simulink model "mamdani_25_rules_trimf_centroid_squarewave"  (R2016b)
settings: Solver=ode45  StartTime=0.0  StopTime=1000  RelTol=1e-3  EnableMultiTasking=on
libraries: fuzblock x1
settings Model: ModifiedByFormat=adolfo  Creator=adolfo  LastModifiedBy=adolfo
settings SolverCC: ZeroCrossControl=DisableAll  ZeroCrossAlgorithm=Adaptive
settings DataIOCC: LimitDataPoints=on  SaveFormat=Array
settings OptimizationCC: LifeSpan=inf
settings DebuggingCC: SolverPrmCheckMsg=warning  SFUnexpectedBacktrackingDiag=warning  SFNoUnconditionalDefaultTransitionDiag=warning  SFExecutionAtInitializationDiag=none
settings HardwareCC: ProdBitPerPointer=32  ProdBitPerSizeT=32  ProdBitPerPtrDiffT=32  ProdLargestAtomicFloat=None  ProdIntDivRoundTo=Undefined  ProdEndianess=Unspecified  ProdWordSize=32  ProdHWDeviceType=32-bit Generic
settings ModelReferenceCC: PropagateSignalLabelsOutOfModel=off
settings GRTTargetCC: TargetLangStandard=C89/C90 (ANSI)  GeneratePreprocessorConditionals=Disable all
settings ConfigComp: CovMetricSettings=dw  CovHtmlReporting=on  CovSaveCumulativeToWorkspaceVar=on  CovSaveSingleToWorkspaceVar=on  CovExternalEMLEnable=off  CovSFcnEnable=off

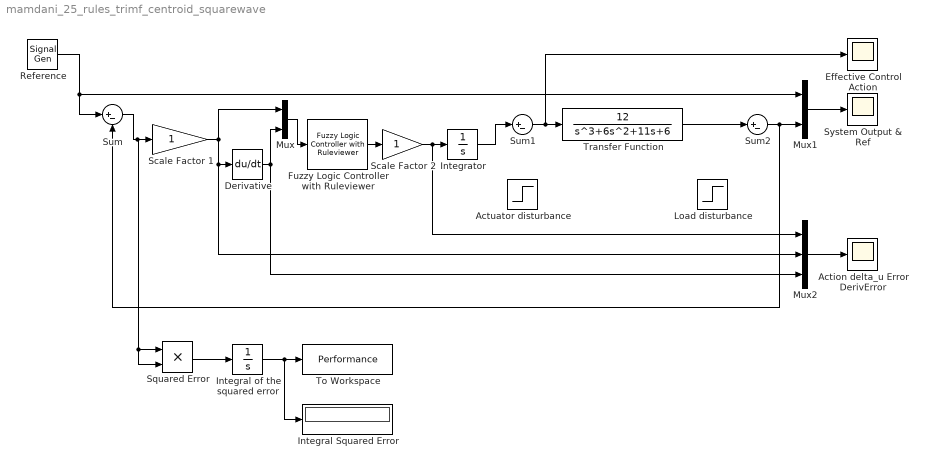
== system mamdani_25_rules_trimf_centroid_squarewave ==
  Action delta_u Error DerivError : Scope
  "Actuator disturbance " : Step  SampleTime=0
  Derivative : Derivative
  "Effective Control Action " : Scope
  Fuzzy Logic Controller with Ruleviewer : fuzblock/Fuzzy Logic  Controller  with Ruleviewer  fismatrix=mamdani_25_rules_trimf_centroid  Ts=1
  "Integral Squared Error " : Display
  "Integral of the squared error " : Integrator
  Integrator : Integrator
  Load disturbance : Step  SampleTime=0
  Mux : Mux  Inputs=2
  Mux1 : Mux  Inputs=2
  Mux2 : Mux  Inputs=3
  Reference : SignalGenerator  WaveForm=square  Amplitude=-1  Frequency=0.01  Units=rad/sec
  Scale Factor 1 : Gain
  Scale Factor 2 : Gain
  Squared Error : Product
  Sum : Sum  Inputs=|+-
  Sum1 : Sum  Inputs=|+-
  Sum2 : Sum  Inputs=|+-
  System Output & Ref : Scope
  To Workspace : ToWorkspace  VariableName=Performance  SaveFormat=Timeseries  SampleTime=-1
  Transfer Function : TransferFcn  Numerator=[12]  Denominator=[1 6 11 6]
  wires:
  Reference/1 -> Sum/1, Mux1/1
  Sum/1 -> Squared Error/2, Squared Error/1, Scale Factor 1/1
  Derivative/1 -> Mux2/3, Mux/2
  Scale Factor 1/1 -> Mux/1, Mux2/2, Derivative/1
  Scale Factor 2/1 -> Mux2/1, Integrator/1
  Integrator/1 -> Sum1/1
  Sum1/1 -> "Effective Control Action "/1, Transfer Function/1
  Transfer Function/1 -> Sum2/1
  Sum2/1 -> Sum/2, Mux1/2
  Mux1/1 -> System Output & Ref/1
  Mux2/1 -> Action delta_u Error DerivError/1
  Squared Error/1 -> "Integral of the squared error "/1
  "Integral of the squared error "/1 -> "Integral Squared Error "/1, To Workspace/1
  Fuzzy Logic Controller with Ruleviewer/1 -> Scale Factor 2/1
  Mux/1 -> Fuzzy Logic Controller with Ruleviewer/1
